simulink model "part2_5"  (R2023b)
settings: Solver=VariableStepAuto  StartTime=0.0  StopTime=10.0  RelTol=1e-3
settings Model: Creator=Zahedi  LastModifiedBy=Zahedi

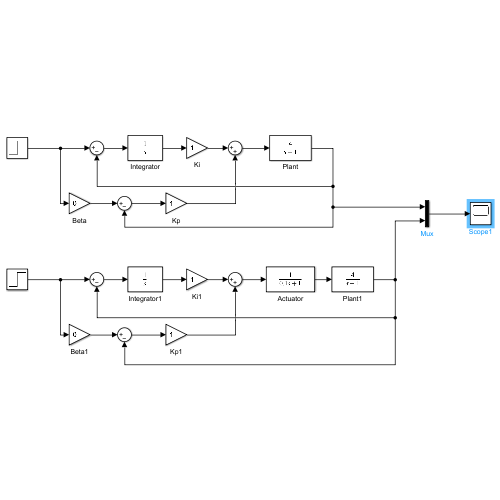
[thumbnail: Simulink's stored preview of the top-level diagram]
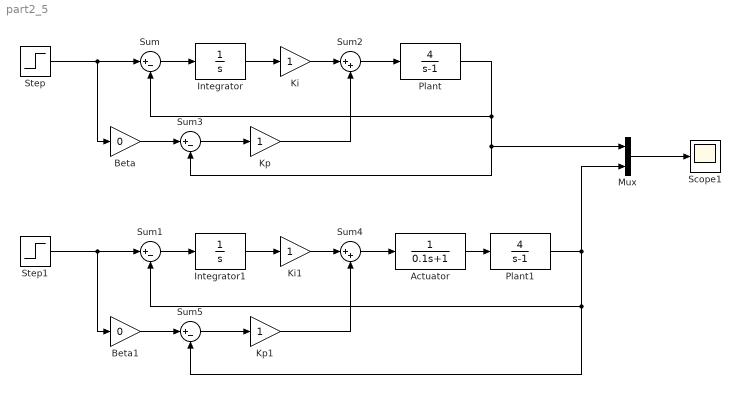
== system part2_5 ==
  Actuator : TransferFcn  Denominator=[0.1 1]
  Beta : Gain  Gain=0
  Beta1 : Gain  Gain=0
  Integrator : TransferFcn  Denominator=[1 0]
  Integrator1 : TransferFcn  Denominator=[1 0]
  Ki : Gain
  Ki1 : Gain
  Kp : Gain
  Kp1 : Gain
  Mux : Mux  Inputs=2
  Plant : TransferFcn  Numerator=[4]  Denominator=[1 -1]
  Plant1 : TransferFcn  Numerator=[4]  Denominator=[1 -1]
  Scope1 : Scope
  Step : Step  SampleTime=0
  Step1 : Step  SampleTime=0
  Sum{,1,3,5} (4 alike) : Sum  Inputs=|+-
  Sum2 : Sum  Inputs=|++
  Sum4 : Sum  Inputs=|++
  wires:
  Plant/1 -> Mux/1, Sum3/2, Sum/2
  Sum/1 -> Integrator/1
  Step/1 -> Beta/1, Sum/1
  Sum2/1 -> Plant/1
  Beta/1 -> Sum3/1
  Kp/1 -> Sum2/2
  Sum3/1 -> Kp/1
  Ki/1 -> Sum2/1
  Integrator/1 -> Ki/1
  Kp1/1 -> Sum4/2
  Ki1/1 -> Sum4/1
  Sum5/1 -> Kp1/1
  Integrator1/1 -> Ki1/1
  Sum1/1 -> Integrator1/1
  Beta1/1 -> Sum5/1
  Step1/1 -> Beta1/1, Sum1/1
  Plant1/1 -> Sum5/2, Sum1/2, Mux/2
  Actuator/1 -> Plant1/1
  Sum4/1 -> Actuator/1
  Mux/1 -> Scope1/1
